simulink model "Cart_Pole_Simulink_Test"  (R2021b)
settings: Solver=VariableStepAuto  StartTime=0.0  StopTime=2  RelTol=1e-3
PreLoadFcn:
  | l =1;
  | mp = 1;
  | mc = 1;
  | g = 10;
values from neighbouring files (symbols this model uses):
  K = place(A,B,lambda)    [state_space_cartpole_simulink.m]
settings Model: Creator=mithu  LastModifiedBy=mithu

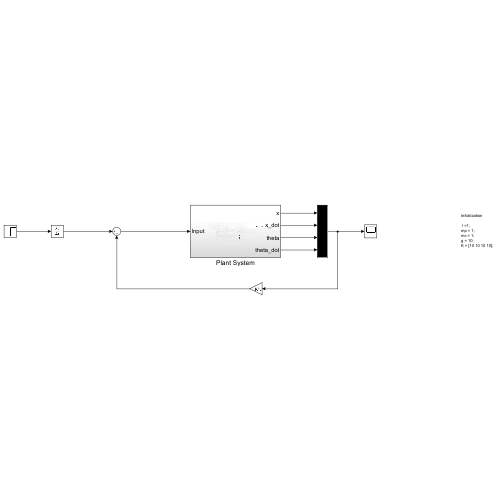
[thumbnail: Simulink's stored preview of the top-level diagram]
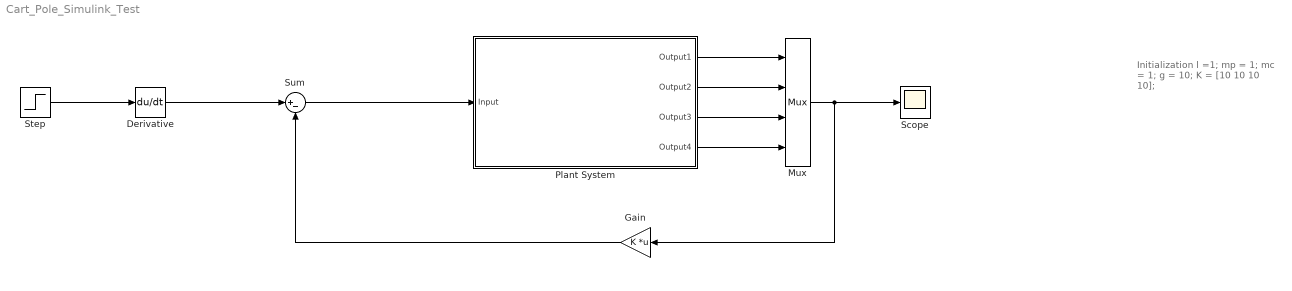
== system Cart_Pole_Simulink_Test ==
  note: Initialization
      |
      |  l =1;
      | mp = 1;
      | mc = 1;
      | g = 10;
      | K = [10 10 10 10];
  Derivative : Derivative
  Gain : Gain  Gain=K  Multiplication=Matrix(K*u)
  Mux : Mux
  Plant System : Subsystem
  Scope : Scope
  Step : Step  Time=0.0001  SampleTime=0
  Sum : Sum  Inputs=|+-
  wires:
  Mux/1 -> Scope/1, Gain/1
  Plant System/1(Output1) -> Mux/1
  Plant System/2(Output2) -> Mux/2
  Plant System/3(Output3) -> Mux/3
  Plant System/4(Output4) -> Mux/4
  Gain/1 -> Sum/2
  Sum/1 -> Plant System/1(Input)
  Step/1 -> Derivative/1
  Derivative/1 -> Sum/1

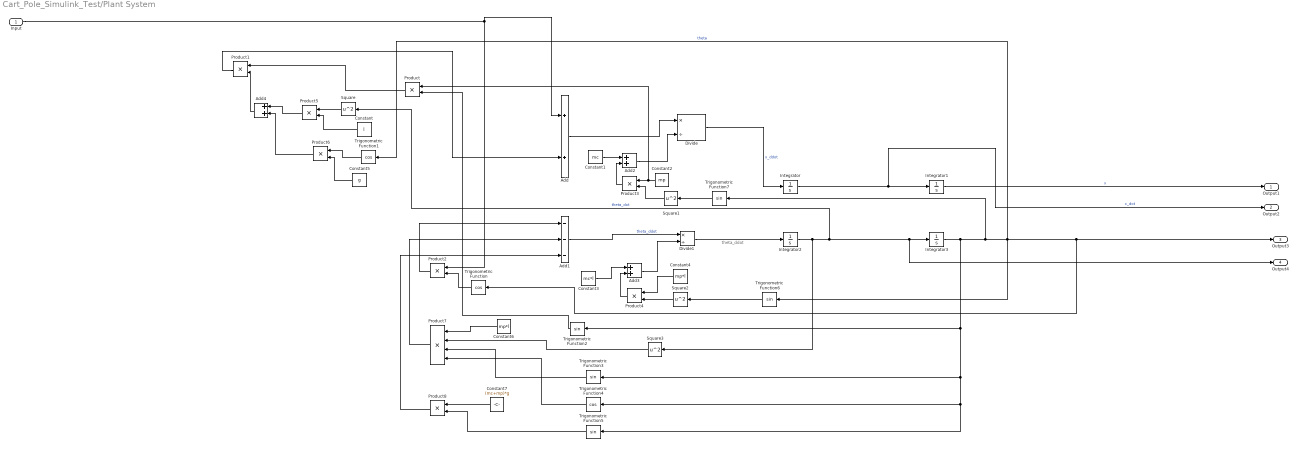
== system Cart_Pole_Simulink_Test/Plant System ==
  note: theta_ddot
  Input : Inport
  Add{,2..4} (4 alike) : Sum
  Add1 : Sum  Inputs=---
  Constant : Constant  Value=l
  Constant1 : Constant  Value=mc
  Constant2 : Constant  Value=mp
  Constant3 : Constant  Value=mc*l
  Constant4 : Constant  Value=mp*l
  Constant5 : Constant  Value=g
  Constant6 : Constant  Value=mp*l
  Constant7 : Constant  Value=(mc+mp)*g
  Divide : Product  Inputs=*/
  Divide1 : Product  Inputs=*/
  Integrator{,1..3} (4 alike) : Integrator
  Product{,1..6,8} (8 alike) : Product
  Product7 : Product  Inputs=4
  Square{,1..3} (4 alike) : Math  Operator=square  SaturateOnIntegerOverflow=on
  Trigonometric Function : Trigonometry  Operator=cos
  Trigonometric Function1 : Trigonometry  Operator=cos
  Trigonometric Function{2..3,5..7} (5 alike) : Trigonometry
  Trigonometric Function4 : Trigonometry  Operator=cos
  Output1 : Outport
  Output2 : Outport  Port=2
  Output3 : Outport  Port=3
  Output4 : Outport  Port=4
  wires:
  Integrator3/1 -> Trigonometric Function7/1, Trigonometric Function6/1, Trigonometric Function1/1, Output3/1, Trigonometric Function/1, Trigonometric Function5/1, Trigonometric Function4/1, Trigonometric Function3/1, Trigonometric Function2/1  "theta"
  Divide/1 -> Integrator/1  "x_ddot"
  Integrator/1 -> Output2/1, Integrator1/1  "x_dot"
  Trigonometric Function5/1 -> Product8/2
  Integrator1/1 -> Output1/1  "x"
  Integrator2/1 -> Square3/1, Square/1, Output4/1, Integrator3/1  "theta_dot"
  Square2/1 -> Product4/2
  Product5/1 -> Add4/1
  Product8/1 -> Add1/3
  Input/1 -> Add/1, Product2/1
  Add/1 -> Divide/1
  Product3/1 -> Add2/2
  Square/1 -> Product5/1
  Product7/1 -> Add1/2
  Product4/1 -> Add3/2
  Product1/1 -> Add/2
  Constant3/1 -> Add3/1
  Product6/1 -> Add4/2
  Constant/1 -> Product5/2
  Constant1/1 -> Add2/1
  Product/1 -> Product1/1
  Constant2/1 -> Product/1, Product3/1
  Square1/1 -> Product3/2
  Trigonometric Function3/1 -> Product7/3
  Add2/1 -> Divide/2
  Add4/1 -> Product1/2
  Constant4/1 -> Product4/1
  Constant7/1 -> Product8/1
  Product2/1 -> Add1/1
  Trigonometric Function4/1 -> Product7/4
  Constant6/1 -> Product7/1
  Trigonometric Function/1 -> Product2/2
  Trigonometric Function1/1 -> Product6/1
  Trigonometric Function2/1 -> Product/2
  Constant5/1 -> Product6/2
  Square3/1 -> Product7/2
  Add3/1 -> Divide1/2
  Trigonometric Function6/1 -> Square2/1
  Divide1/1 -> Integrator2/1
  Add1/1 -> Divide1/1  "theta_ddot"
  Trigonometric Function7/1 -> Square1/1
